simulink model "SPI_controller_interface"  (R2015a)
settings: Solver=FixedStepDiscrete  StartTime=0.0  StopTime=inf  FixedStep=ts  RelTol=1e-3
model workspace (MAT data in the model file):
  message_length = Simulink.Parameter
  message_length.Value = 16
  message_length.DataType = 'uint16'
  clk_freq = Simulink.Parameter
  clk_freq.Value = 1000000
  clk_freq.DataType = 'uint32'
  cs_to_clk_edge = Simulink.Parameter
  cs_to_clk_edge.Value = 35
  cs_to_clk_edge.DataType = 'uint16'
  stall_time = Simulink.Parameter
  stall_time.Value = 4
  stall_time.DataType = 'uint16'
undefined symbols (not defined in the file): AXI4, Lite
libraries: axiinterfacelib x14
settings Model: SimulationMode=external  CovSFcnEnable=off  Creator=bsoheili  LastModifiedBy=dlwalter
settings DataIOCC: SaveOutput=off  SaveTime=off
settings OptimizationCC: BlockReduction=off  ConditionallyExecuteInputs=off  UseDivisionForNetSlopeComputation=UseDivisionForReciprocalsOfIntegersOnly  UseFloatMulNetSlope=on  EnhancedBackFolding=on  EfficientFloat2IntCast=on  OptimizeModelRefInitCode=on  LifeSpan=1  MaxStackSize=64
settings DebuggingCC: AlgebraicLoopMsg=error  SolverPrmCheckMsg=warning  InheritedTsInSrcMsg=none  StrictBusMsg=ErrorOnBusTreatedAsVector  NonBusSignalsTreatedAsBus=error
settings HardwareCC: ProdLargestAtomicInteger=Long  ProdLargestAtomicFloat=Double  ProdEndianess=LittleEndian  ProdHWDeviceType=ARM Compatible->ARM Cortex  ProdEqTarget=off
settings RTWCC: SystemTargetFile=ert.tlc  TLCOptions=-aInlineSetEventsForThisBaseRateFcn=TLC_FALSE -aSuppressMultiTaskScheduler=TLC_FALSE  TemplateMakefile=ert_default_tmf  Description=Embedded Coder  GenerateReport=on  Toolchain=Xilinx Software Development Kit (SDK) 2013.4  IncludeHyperlinkInReport=on  LaunchReport=on  GenerateTraceInfo=on  GenerateTraceReport=on  GenerateTraceReportSl=on  GenerateTraceReportSf=on  GenerateTraceReportEml=on  GenerateCodeMetricsReport=on
settings CodeAppCC: IgnoreCustomStorageClasses=off
settings ERTTargetCC: GenerateSampleERTMain=off  ParMdlRefBuildCompliant=on  CompOptLevelCompliant=on  ConcurrentExecutionCompliant=on  CombineSignalStateStructs=on  ERTFirstTimeCompliant=on  SupportContinuousTime=off  SupportVariableSizeSignals=off  ModelStepFunctionPrototypeControlCompliant=on  CPPClassGenCompliant=on

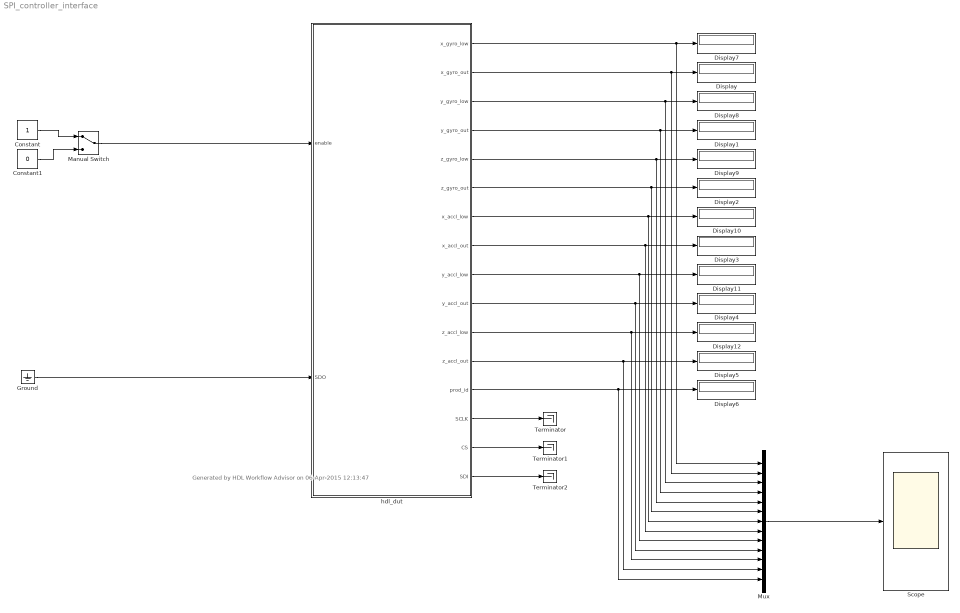
== system SPI_controller_interface ==
  note: Generated by HDL Workflow Advisor on 06-Apr-2015 12:13:47
  Constant : Constant  OutDataTypeStr=boolean  SampleTime=-1
  Constant1 : Constant  Value=0  OutDataTypeStr=boolean  SampleTime=-1
  Display{,1..12} (13 alike) : Display
  Ground : Ground
  Manual Switch : ManualSwitch
  Mux : Mux  Inputs=13
  Scope : Scope
      settings: TimeRange=1  YMin=-35000  YMax=35000
  Terminator : Terminator
  Terminator1 : Terminator
  Terminator2 : Terminator
  hdl_dut : Subsystem  TreatAsAtomicUnit=on  MinMaxOverflowLogging=MinMaxAndOverflow  mask(AXI4-Lite/AXI4 Interface){}
      mask help:
      | This is an automatically generated subsystem block.
      | This contains the AXI4-Lite/AXI4 interface which communicates with the SPI_controller_PL_only_Subsystem_ipcore IPCore generated from SPI_controller_PL_only/hdl_dut subsystem.
      mask Display: disp(sprintf('Xilinx Zynq \nAXI4-Lite/AXI4 Interface'));
  wires:
  hdl_dut/12(z_accl_out) -> Mux/12, Display5/1
  hdl_dut/10(y_accl_out) -> Mux/10, Display4/1
  hdl_dut/6(z_gyro_out) -> Mux/6, Display2/1
  hdl_dut/4(y_gyro_out) -> Mux/4, Display1/1
  hdl_dut/2(x_gyro_out) -> Mux/2, Display/1
  Ground/1 -> hdl_dut/2(SDO)
  Manual Switch/1 -> hdl_dut/1(enable)
  hdl_dut/14(SCLK) -> Terminator/1
  hdl_dut/15(CS) -> Terminator1/1
  hdl_dut/16(SDI) -> Terminator2/1
  hdl_dut/13(prod_id) -> Mux/13, Display6/1
  hdl_dut/1(x_gyro_low) -> Mux/1, Display7/1
  hdl_dut/3(y_gyro_low) -> Mux/3, Display8/1
  hdl_dut/7(x_accl_low) -> Mux/7, Display10/1
  hdl_dut/5(z_gyro_low) -> Mux/5, Display9/1
  hdl_dut/9(y_accl_low) -> Mux/9, Display11/1
  hdl_dut/11(z_accl_low) -> Mux/11, Display12/1
  Constant/1 -> Manual Switch/1
  Constant1/1 -> Manual Switch/2
  hdl_dut/8(x_accl_out) -> Mux/8, Display3/1
  Mux/1 -> Scope/1

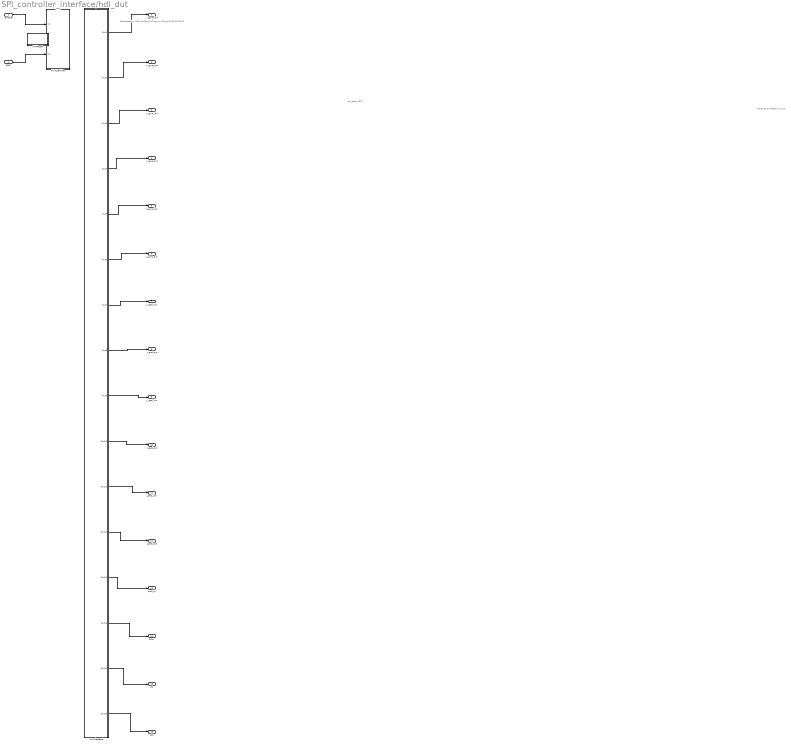
== system SPI_controller_interface/hdl_dut ==
  note: spi_read_ADIS
  note: Assigned to PMOD pins out
  note: Generated by HDL Workflow Advisor on 06-Apr-2015 15:03:23
  enable : Inport
  SDO : Inport  Port=2
  AXI4LiteRead : Subsystem  Priority=10
  AXI4LiteWrite : Subsystem  Priority=1
  AXI4Reset : Subsystem  mask(System Initialize){ShowInLibBrowser=0}
      mask prompts: ShowInLibBrowser "Simulink:masks:CustCodeMaskParam1_MP"
      settings: CopyFcn=cccopyfcn(gcb)  OpenFcn=ccopenfcn('System Initialize Function')
      mask Help: eval('feval(''rtwprivate'',''rtwhelpview'',''rtw_sys_initialize_block'')');
      mask Display: disp('System\nInitialize');
  x_gyro_low : Outport
  x_gyro_out : Outport  Port=2
  y_gyro_low : Outport  Port=3
  y_gyro_out : Outport  Port=4
  z_gyro_low : Outport  Port=5
  z_gyro_out : Outport  Port=6
  x_accl_low : Outport  Port=7
  x_accl_out : Outport  Port=8
  y_accl_low : Outport  Port=9
  y_accl_out : Outport  Port=10
  z_accl_low : Outport  Port=11
  z_accl_out : Outport  Port=12
  prod_id : Outport  Port=13
  SCLK : Outport  Port=14
  CS : Outport  Port=15
  SDI : Outport  Port=16
  wires:
  enable/1 -> AXI4LiteWrite/1(In1)
  SDO/1 -> AXI4LiteWrite/2(In2)
  AXI4LiteRead/1(Out1) -> x_gyro_low/1
  AXI4LiteRead/2(Out2) -> x_gyro_out/1
  AXI4LiteRead/3(Out3) -> y_gyro_low/1
  AXI4LiteRead/4(Out4) -> y_gyro_out/1
  AXI4LiteRead/5(Out5) -> z_gyro_low/1
  AXI4LiteRead/6(Out6) -> z_gyro_out/1
  AXI4LiteRead/7(Out7) -> x_accl_low/1
  AXI4LiteRead/8(Out8) -> x_accl_out/1
  AXI4LiteRead/9(Out9) -> y_accl_low/1
  AXI4LiteRead/10(Out10) -> y_accl_out/1
  AXI4LiteRead/11(Out11) -> z_accl_low/1
  AXI4LiteRead/12(Out12) -> z_accl_out/1
  AXI4LiteRead/13(Out13) -> prod_id/1
  AXI4LiteRead/14(Out14) -> SCLK/1
  AXI4LiteRead/15(Out15) -> CS/1
  AXI4LiteRead/16(Out16) -> SDI/1

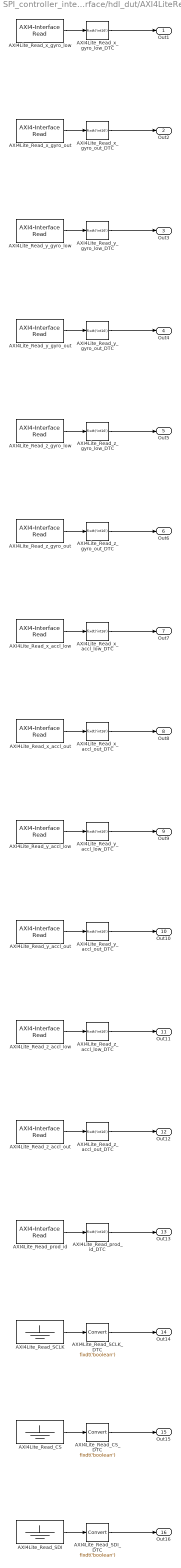
== system SPI_controller_interface/hdl_dut/AXI4LiteRead ==
  AXI4Lite_Read_CS : Ground
  AXI4Lite_Read_CS_DTC : DataTypeConversion  OutDataTypeStr=fixdt('boolean')  ConvertRealWorld=Stored Integer (SI)
  AXI4Lite_Read_SCLK : Ground
  AXI4Lite_Read_SCLK_DTC : DataTypeConversion  OutDataTypeStr=fixdt('boolean')  ConvertRealWorld=Stored Integer (SI)
  AXI4Lite_Read_SDI : Ground
  AXI4Lite_Read_SDI_DTC : DataTypeConversion  OutDataTypeStr=fixdt('boolean')  ConvertRealWorld=Stored Integer (SI)
  AXI4Lite_Read_prod_id : axiinterfacelib/AXI4-Interface Read  Priority=14  AXIInterfaceType=AXI4-Lite  DeviceName=/dev/mwipcore  RegisterOffset=hex2dec('134')  DataLength=4096  DataType=uint32  SampleTime=-1  blockPlatform=ZYNQ  SimulateUsing=Interpreted Execution
  AXI4Lite_Read_prod_id_DTC : DataTypeConversion  OutDataTypeStr=fixdt('int16')  ConvertRealWorld=Stored Integer (SI)
  AXI4Lite_Read_x_accl_low : axiinterfacelib/AXI4-Interface Read  Priority=8  AXIInterfaceType=AXI4-Lite  DeviceName=/dev/mwipcore  RegisterOffset=hex2dec('11C')  DataLength=4096  DataType=uint32  SampleTime=-1  blockPlatform=ZYNQ  SimulateUsing=Interpreted Execution
  AXI4Lite_Read_x_accl_low_DTC : DataTypeConversion  OutDataTypeStr=fixdt('int16')  ConvertRealWorld=Stored Integer (SI)
  AXI4Lite_Read_x_accl_out : axiinterfacelib/AXI4-Interface Read  Priority=9  AXIInterfaceType=AXI4-Lite  DeviceName=/dev/mwipcore  RegisterOffset=hex2dec('120')  DataLength=4096  DataType=uint32  SampleTime=-1  blockPlatform=ZYNQ  SimulateUsing=Interpreted Execution
  AXI4Lite_Read_x_accl_out_DTC : DataTypeConversion  OutDataTypeStr=fixdt('int16')  ConvertRealWorld=Stored Integer (SI)
  AXI4Lite_Read_x_gyro_low : axiinterfacelib/AXI4-Interface Read  Priority=2  AXIInterfaceType=AXI4-Lite  DeviceName=/dev/mwipcore  RegisterOffset=hex2dec('104')  DataLength=4096  DataType=uint32  SampleTime=-1  blockPlatform=ZYNQ  SimulateUsing=Interpreted Execution
  AXI4Lite_Read_x_gyro_low_DTC : DataTypeConversion  OutDataTypeStr=fixdt('int16')  ConvertRealWorld=Stored Integer (SI)
  AXI4Lite_Read_x_gyro_out : axiinterfacelib/AXI4-Interface Read  Priority=3  AXIInterfaceType=AXI4-Lite  DeviceName=/dev/mwipcore  RegisterOffset=hex2dec('108')  DataLength=4096  DataType=uint32  SampleTime=-1  blockPlatform=ZYNQ  SimulateUsing=Interpreted Execution
  AXI4Lite_Read_x_gyro_out_DTC : DataTypeConversion  OutDataTypeStr=fixdt('int16')  ConvertRealWorld=Stored Integer (SI)
  AXI4Lite_Read_y_accl_low : axiinterfacelib/AXI4-Interface Read  Priority=10  AXIInterfaceType=AXI4-Lite  DeviceName=/dev/mwipcore  RegisterOffset=hex2dec('124')  DataLength=4096  DataType=uint32  SampleTime=-1  blockPlatform=ZYNQ  SimulateUsing=Interpreted Execution
  AXI4Lite_Read_y_accl_low_DTC : DataTypeConversion  OutDataTypeStr=fixdt('int16')  ConvertRealWorld=Stored Integer (SI)
  AXI4Lite_Read_y_accl_out : axiinterfacelib/AXI4-Interface Read  Priority=11  AXIInterfaceType=AXI4-Lite  DeviceName=/dev/mwipcore  RegisterOffset=hex2dec('128')  DataLength=4096  DataType=uint32  SampleTime=-1  blockPlatform=ZYNQ  SimulateUsing=Interpreted Execution
  AXI4Lite_Read_y_accl_out_DTC : DataTypeConversion  OutDataTypeStr=fixdt('int16')  ConvertRealWorld=Stored Integer (SI)
  AXI4Lite_Read_y_gyro_low : axiinterfacelib/AXI4-Interface Read  Priority=4  AXIInterfaceType=AXI4-Lite  DeviceName=/dev/mwipcore  RegisterOffset=hex2dec('10C')  DataLength=4096  DataType=uint32  SampleTime=-1  blockPlatform=ZYNQ  SimulateUsing=Interpreted Execution
  AXI4Lite_Read_y_gyro_low_DTC : DataTypeConversion  OutDataTypeStr=fixdt('int16')  ConvertRealWorld=Stored Integer (SI)
  AXI4Lite_Read_y_gyro_out : axiinterfacelib/AXI4-Interface Read  Priority=5  AXIInterfaceType=AXI4-Lite  DeviceName=/dev/mwipcore  RegisterOffset=hex2dec('110')  DataLength=4096  DataType=uint32  SampleTime=-1  blockPlatform=ZYNQ  SimulateUsing=Interpreted Execution
  AXI4Lite_Read_y_gyro_out_DTC : DataTypeConversion  OutDataTypeStr=fixdt('int16')  ConvertRealWorld=Stored Integer (SI)
  AXI4Lite_Read_z_accl_low : axiinterfacelib/AXI4-Interface Read  Priority=12  AXIInterfaceType=AXI4-Lite  DeviceName=/dev/mwipcore  RegisterOffset=hex2dec('12C')  DataLength=4096  DataType=uint32  SampleTime=-1  blockPlatform=ZYNQ  SimulateUsing=Interpreted Execution
  AXI4Lite_Read_z_accl_low_DTC : DataTypeConversion  OutDataTypeStr=fixdt('int16')  ConvertRealWorld=Stored Integer (SI)
  AXI4Lite_Read_z_accl_out : axiinterfacelib/AXI4-Interface Read  Priority=13  AXIInterfaceType=AXI4-Lite  DeviceName=/dev/mwipcore  RegisterOffset=hex2dec('130')  DataLength=4096  DataType=uint32  SampleTime=-1  blockPlatform=ZYNQ  SimulateUsing=Interpreted Execution
  AXI4Lite_Read_z_accl_out_DTC : DataTypeConversion  OutDataTypeStr=fixdt('int16')  ConvertRealWorld=Stored Integer (SI)
  AXI4Lite_Read_z_gyro_low : axiinterfacelib/AXI4-Interface Read  Priority=6  AXIInterfaceType=AXI4-Lite  DeviceName=/dev/mwipcore  RegisterOffset=hex2dec('114')  DataLength=4096  DataType=uint32  SampleTime=-1  blockPlatform=ZYNQ  SimulateUsing=Interpreted Execution
  AXI4Lite_Read_z_gyro_low_DTC : DataTypeConversion  OutDataTypeStr=fixdt('int16')  ConvertRealWorld=Stored Integer (SI)
  AXI4Lite_Read_z_gyro_out : axiinterfacelib/AXI4-Interface Read  Priority=7  AXIInterfaceType=AXI4-Lite  DeviceName=/dev/mwipcore  RegisterOffset=hex2dec('118')  DataLength=4096  DataType=uint32  SampleTime=-1  blockPlatform=ZYNQ  SimulateUsing=Interpreted Execution
  AXI4Lite_Read_z_gyro_out_DTC : DataTypeConversion  OutDataTypeStr=fixdt('int16')  ConvertRealWorld=Stored Integer (SI)
  Out1 : Outport
  Out2 : Outport  Port=2
  Out3 : Outport  Port=3
  Out4 : Outport  Port=4
  Out5 : Outport  Port=5
  Out6 : Outport  Port=6
  Out7 : Outport  Port=7
  Out8 : Outport  Port=8
  Out9 : Outport  Port=9
  Out10 : Outport  Port=10
  Out11 : Outport  Port=11
  Out12 : Outport  Port=12
  Out13 : Outport  Port=13
  Out14 : Outport  Port=14
  Out15 : Outport  Port=15
  Out16 : Outport  Port=16
  wires:
  AXI4Lite_Read_SDI_DTC/1 -> Out16/1
  AXI4Lite_Read_SDI/1 -> AXI4Lite_Read_SDI_DTC/1
  AXI4Lite_Read_CS_DTC/1 -> Out15/1
  AXI4Lite_Read_CS/1 -> AXI4Lite_Read_CS_DTC/1
  AXI4Lite_Read_SCLK_DTC/1 -> Out14/1
  AXI4Lite_Read_SCLK/1 -> AXI4Lite_Read_SCLK_DTC/1
  AXI4Lite_Read_prod_id/1 -> AXI4Lite_Read_prod_id_DTC/1
  AXI4Lite_Read_prod_id_DTC/1 -> Out13/1
  AXI4Lite_Read_z_accl_out/1 -> AXI4Lite_Read_z_accl_out_DTC/1
  AXI4Lite_Read_z_accl_out_DTC/1 -> Out12/1
  AXI4Lite_Read_z_accl_low/1 -> AXI4Lite_Read_z_accl_low_DTC/1
  AXI4Lite_Read_z_accl_low_DTC/1 -> Out11/1
  AXI4Lite_Read_y_accl_out/1 -> AXI4Lite_Read_y_accl_out_DTC/1
  AXI4Lite_Read_y_accl_out_DTC/1 -> Out10/1
  AXI4Lite_Read_y_accl_low/1 -> AXI4Lite_Read_y_accl_low_DTC/1
  AXI4Lite_Read_y_accl_low_DTC/1 -> Out9/1
  AXI4Lite_Read_x_accl_out/1 -> AXI4Lite_Read_x_accl_out_DTC/1
  AXI4Lite_Read_x_accl_out_DTC/1 -> Out8/1
  AXI4Lite_Read_x_accl_low/1 -> AXI4Lite_Read_x_accl_low_DTC/1
  AXI4Lite_Read_x_accl_low_DTC/1 -> Out7/1
  AXI4Lite_Read_z_gyro_out/1 -> AXI4Lite_Read_z_gyro_out_DTC/1
  AXI4Lite_Read_z_gyro_out_DTC/1 -> Out6/1
  AXI4Lite_Read_z_gyro_low/1 -> AXI4Lite_Read_z_gyro_low_DTC/1
  AXI4Lite_Read_z_gyro_low_DTC/1 -> Out5/1
  AXI4Lite_Read_y_gyro_out/1 -> AXI4Lite_Read_y_gyro_out_DTC/1
  AXI4Lite_Read_y_gyro_out_DTC/1 -> Out4/1
  AXI4Lite_Read_y_gyro_low/1 -> AXI4Lite_Read_y_gyro_low_DTC/1
  AXI4Lite_Read_y_gyro_low_DTC/1 -> Out3/1
  AXI4Lite_Read_x_gyro_low_DTC/1 -> Out1/1
  AXI4Lite_Read_x_gyro_low/1 -> AXI4Lite_Read_x_gyro_low_DTC/1
  AXI4Lite_Read_x_gyro_out/1 -> AXI4Lite_Read_x_gyro_out_DTC/1
  AXI4Lite_Read_x_gyro_out_DTC/1 -> Out2/1

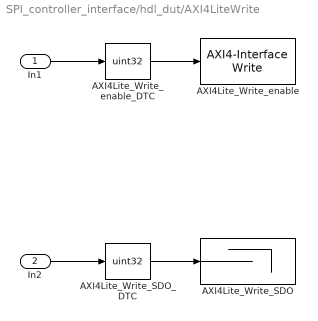
== system SPI_controller_interface/hdl_dut/AXI4LiteWrite ==
  In1 : Inport
  In2 : Inport  Port=2
  AXI4Lite_Write_SDO : Terminator
  AXI4Lite_Write_SDO_DTC : DataTypeConversion  OutDataTypeStr=uint32  ConvertRealWorld=Stored Integer (SI)
  AXI4Lite_Write_enable : axiinterfacelib/AXI4-Interface Write  Priority=1  AXIInterfaceType=AXI4-Lite  DeviceName=/dev/mwipcore  RegisterOffset=hex2dec('100')  blockPlatform=ZYNQ  SimulateUsing=Interpreted execution
  AXI4Lite_Write_enable_DTC : DataTypeConversion  OutDataTypeStr=uint32  ConvertRealWorld=Stored Integer (SI)
  wires:
  AXI4Lite_Write_SDO_DTC/1 -> AXI4Lite_Write_SDO/1
  In2/1 -> AXI4Lite_Write_SDO_DTC/1
  In1/1 -> AXI4Lite_Write_enable_DTC/1
  AXI4Lite_Write_enable_DTC/1 -> AXI4Lite_Write_enable/1

== system SPI_controller_interface/hdl_dut/AXI4Reset ==
